simulink model "Magic_tire_model"  (R2022b)
settings: Solver=VariableStepAuto  StartTime=0.0  StopTime=sim_time  RelTol=1e-3
libraries: simulink x2
settings Model: Creator=FATMANURATA  LastModifiedBy=FATMANURATA

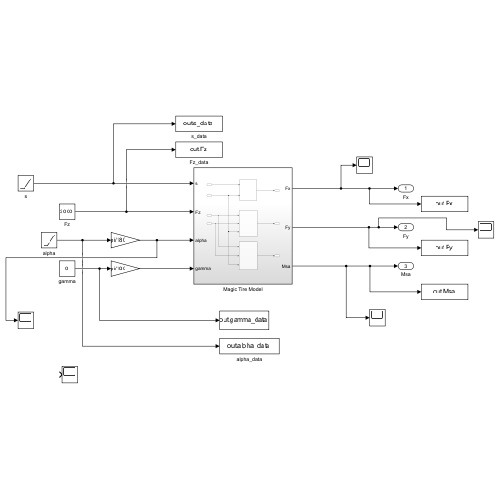
[thumbnail: Simulink's stored preview of the top-level diagram]
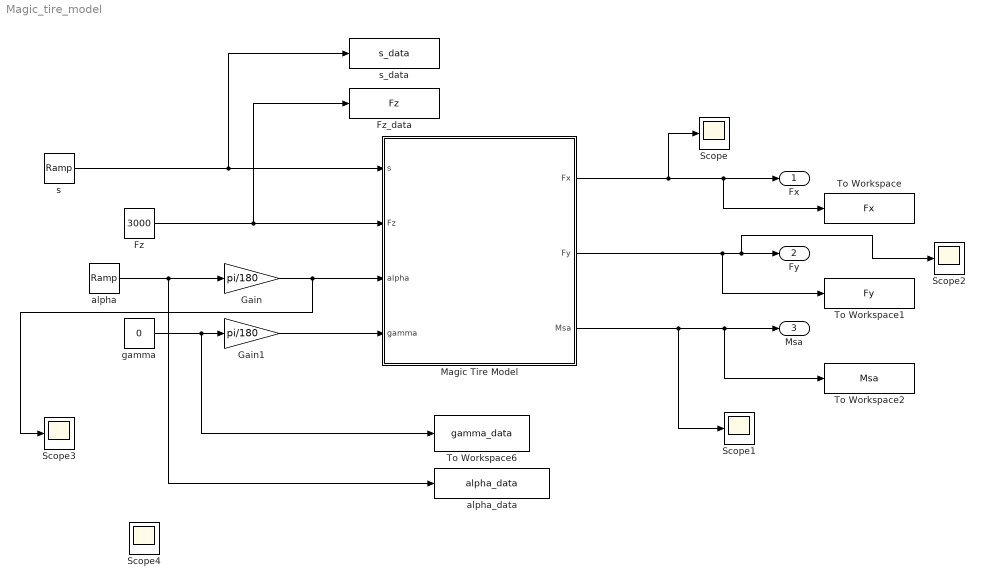
== system Magic_tire_model ==
  Fz : Constant  Value=3000
  Fz_data : ToWorkspace  VariableName=Fz  SaveFormat=Structure With Time  SampleTime=-1
  Gain : Gain  Gain=pi/180
  Gain1 : Gain  Gain=pi/180
  Magic Tire Model : Subsystem
  Scope{,1..4} (5 alike) : Scope
  To Workspace : ToWorkspace  VariableName=Fx  SaveFormat=Structure With Time  SampleTime=-1
  To Workspace1 : ToWorkspace  VariableName=Fy  SaveFormat=Structure With Time  SampleTime=-1
  To Workspace2 : ToWorkspace  VariableName=Msa  SaveFormat=Structure With Time  SampleTime=-1
  To Workspace6 : ToWorkspace  VariableName=gamma_data  SaveFormat=Structure With Time  SampleTime=-1
  alpha : simulink/Sources/Ramp  slope=3  start=0  InitialOutput=-300
  alpha_data : ToWorkspace  VariableName=alpha_data  SaveFormat=Structure With Time  SampleTime=-1
  gamma : Constant  Value=0
  s : simulink/Sources/Ramp  slope=1  start=0  InitialOutput=-100
  s_data : ToWorkspace  VariableName=s_data  SaveFormat=Structure With Time  SampleTime=-1
  Fx : Outport
  Fy : Outport  Port=2
  Msa : Outport  Port=3
  wires:
  Fz/1 -> Fz_data/1, Magic Tire Model/2(Fz)
  Magic Tire Model/3(Msa) -> Scope1/1, To Workspace2/1, Msa/1
  Gain/1 -> Magic Tire Model/3(alpha), Scope3/1
  gamma/1 -> Gain1/1, To Workspace6/1
  Magic Tire Model/2(Fy) -> To Workspace1/1, Scope2/1, Fy/1
  Magic Tire Model/1(Fx) -> Scope/1, To Workspace/1, Fx/1
  s/1 -> s_data/1, Magic Tire Model/1(s)
  alpha/1 -> alpha_data/1, Gain/1
  Gain1/1 -> Magic Tire Model/4(gamma)

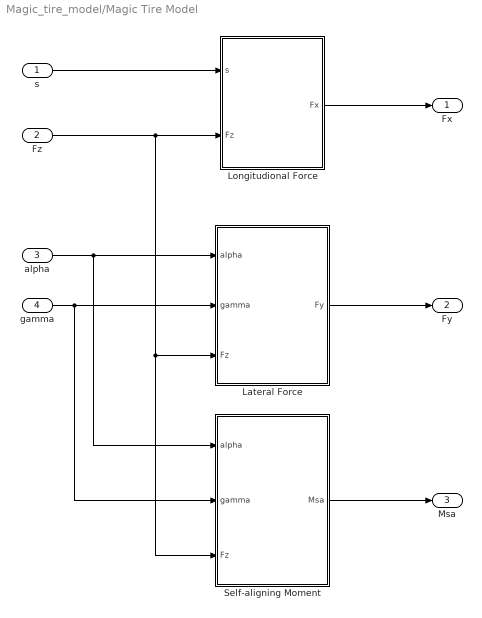
== system Magic_tire_model/Magic Tire Model ==
  s : Inport
  Fz : Inport  Port=2
  alpha : Inport  Port=3
  gamma : Inport  Port=4
  Lateral Force : Subsystem
  Longitudional Force : Subsystem
  Self-aligning Moment : Subsystem
  Fx : Outport
  Fy : Outport  Port=2
  Msa : Outport  Port=3
  wires:
  s/1 -> Longitudional Force/1(s)
  Longitudional Force/1(Fx) -> Fx/1
  Fz/1 -> Self-aligning Moment/3(Fz), Lateral Force/3(Fz), Longitudional Force/2(Fz)
  Lateral Force/1(Fy) -> Fy/1
  alpha/1 -> Self-aligning Moment/1(alpha), Lateral Force/1(alpha)
  gamma/1 -> Lateral Force/2(gamma), Self-aligning Moment/2(gamma)
  Self-aligning Moment/1(Msa) -> Msa/1

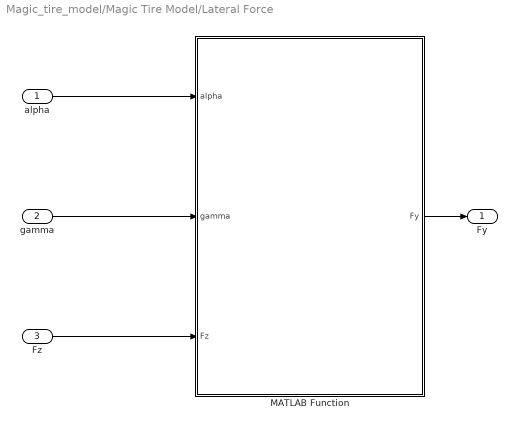
== system Magic_tire_model/Magic Tire Model/Lateral Force ==
  alpha : Inport
  gamma : Inport  Port=2
  Fz : Inport  Port=3
  MATLAB Function : MATLAB Function  TreatAsAtomicUnit=on
  Fy : Outport
  wires:
  alpha/1 -> MATLAB Function/1(alpha)
  MATLAB Function/1(Fy) -> Fy/1
  gamma/1 -> MATLAB Function/2(gamma)
  Fz/1 -> MATLAB Function/3(Fz)

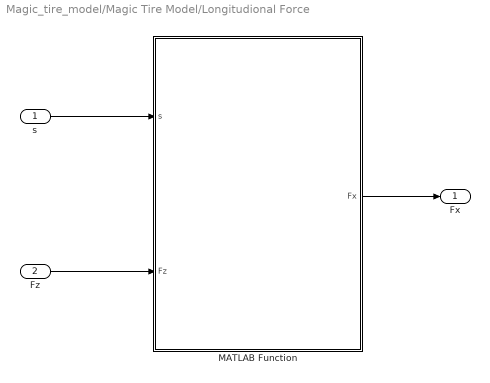
== system Magic_tire_model/Magic Tire Model/Longitudional Force ==
  s : Inport
  Fz : Inport  Port=2
  MATLAB Function : MATLAB Function  TreatAsAtomicUnit=on
  Fx : Outport
  wires:
  s/1 -> MATLAB Function/1(s)
  MATLAB Function/1(Fx) -> Fx/1
  Fz/1 -> MATLAB Function/2(Fz)

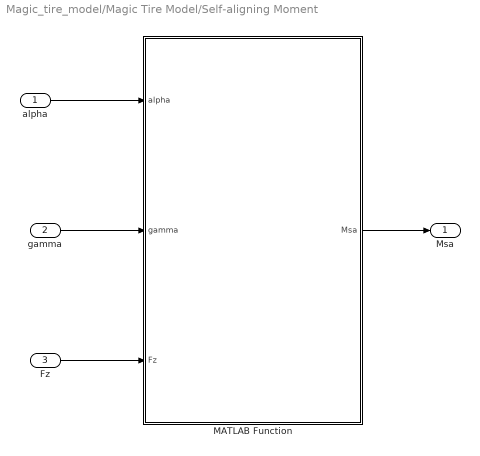
== system Magic_tire_model/Magic Tire Model/Self-aligning Moment ==
  alpha : Inport
  gamma : Inport  Port=2
  Fz : Inport  Port=3
  MATLAB Function : MATLAB Function  TreatAsAtomicUnit=on
  Msa : Outport
  wires:
  Fz/1 -> MATLAB Function/3(Fz)
  alpha/1 -> MATLAB Function/1(alpha)
  gamma/1 -> MATLAB Function/2(gamma)
  MATLAB Function/1(Msa) -> Msa/1

== matlab function Magic_tire_model/Magic Tire Model/Lateral Force/MATLAB Function ==
  data: alpha input; gamma input; Fz input; Fy output
function Fy = fcn(alpha, gamma, Fz)

Fz_kN = Fz / 1000;
% 2. Pacejka Lateral (Fy) Katsayıları 
a0 = 1.6929;
a1 = -55.2084;
a2 = 1271.2800;
a3 = 1601.8000;
a4 = 6.4946;
a5 = 4.7966e-3;
a6 = -0.3875;
a7 = 1.0000;
a8 = -4.5399e-2;
a9 = 4.2832e-3;
a10 = 8.6536e-2;
a11 = -0.2231;
a12 = 7.6680;
a13 = 45.8764;



% Fy için Pacejka Parametrelerinin Hesaplanması 
C = a0;
D = (a1 * Fz_kN + a2) * Fz_kN;
BCD = a3 * sin(2 * atan(Fz_kN / a4)) * (1 - a5 * abs(0)); % Gamma=0 varsayılmıştır
B = BCD / (C * D);
E = a6 * Fz_kN + a7; 
Sh = a8 * gamma + a9 * Fz_kN + a10;
Sv = a11*gamma*Fz_kN + a12*Fz_kN*a13; %Offset removed for clarity
phi = alpha + Sh;

Fy = D * sin(C * atan(B * phi - E * (B * phi - atan(B * phi)))) + Sv;
end

== matlab function Magic_tire_model/Magic Tire Model/Longitudional Force/MATLAB Function ==
  data: s input; Fz input; Fx output
function Fx = fcn(s, Fz)

Fz_kN = Fz / 1000;

% 1. Pacejka Longitudinal (Fx) Katsayıları %from Genta's book
b0 = 1.6500;
b1 = -7.6118;
b2 = 1122.6;
b3 = -7.3600e-3;
b4 = 144.8200;
b5 = -7.6614e-2;
b6 = -3.8600e-3;
b7 = 8.5055e-2;
b8 = 7.5719e-2;
b9 = 2.3655e-2;
b10 = 2.3655e-2;

% Fx için Pacejka Parametrelerinin Hesaplanması 
C = b0; 
D= (b1 * Fz_kN + b2) * Fz_kN;
BCD= (b3 * Fz_kN^2 + b4 * Fz_kN) * exp(-b5 * Fz_kN);
B= BCD/ (C * D);
E= b6 * Fz_kN^2 + b7 * Fz_kN + b8;
Sh= b9 * Fz_kN + b10;
Sv= 0;
phi = s + Sh;

Fx = D * sin(C * atan(B * phi - E * (B * phi - atan(B * phi)))) + Sv;
end

== matlab function Magic_tire_model/Magic Tire Model/Self-aligning Moment/MATLAB Function ==
  data: alpha input; gamma input; Msa output; Fz input

function Msa = fcn(alpha, gamma,Fz)

Fz_kN = Fz / 1000;
c0 = 2.2264;
c1 = -3.0428;
c2 = -9.2284;
c3 = 0.500088;
c4 = -5.56696;
c5 = -0.25964;
c6 = -1.29724e-3;
c7 = -0.358348;
c8 = 3.74476;
c9 = -15.1566;
c10 = 2.1156e-3;
c11 = 3.4600e-4;
c12 = 9.13952e-3;
c13 = -0.244556;
c14 = 0.100695;
c15 = -1.3980;
c16 = 0.44441;
c17 = -0.998344;



C = c0;
D = c1 * Fz_kN^2 + c2 * Fz_kN;
BCD = (c3 * Fz_kN^2 + c4 * Fz_kN) * (1 - c6 * abs(gamma)) * exp(-c5 * Fz_kN);
B = BCD / (C * D);
E = (c7 * Fz_kN^2 + c8 * Fz_kN + c9) * (1 - c10 * abs(gamma));
Sh = c11 * gamma + c12 * Fz_kN + c13;
Sv = (c14 * Fz_kN^2 + c15 * Fz_kN)*gamma + c16 * Fz_kN +c17  ;
phi = alpha + Sh;
Msa = D * sin(C * atan(B * phi - E * (B * phi - atan(B * phi)))) + Sv;
end
